simulink model "Class_task"  (R2020a)
settings: Solver=VariableStepAuto  StartTime=0.0  StopTime=10.0  RelTol=1e-3
settings Model: Creator=User  LastModifiedBy=User

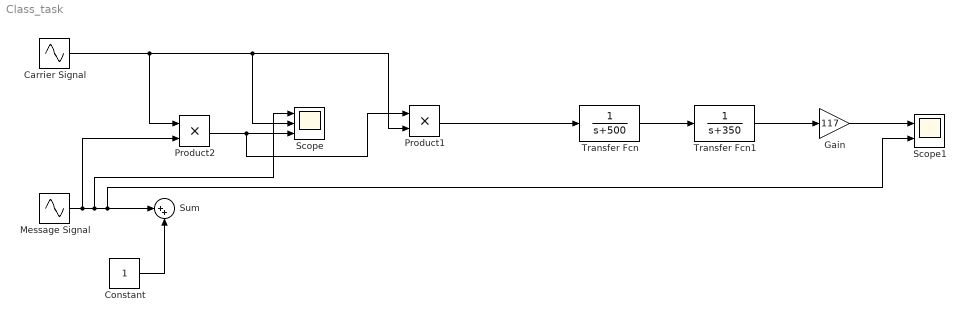
== system Class_task ==
  Carrier Signal : Sin  Amplitude=58  Frequency=2*pi*86  SampleTime=1/5000
  Constant : Constant
  Gain : Gain  Gain=117
  Message Signal : Sin  Amplitude=18  Frequency=2*pi*36  Phase=58  SampleTime=1/5000
  Product1 : Product
  Product2 : Product
  Scope : Scope  NumInputPorts=3
  Scope1 : Scope  NumInputPorts=2
  Sum : Sum  Inputs=|++
  Transfer Fcn : TransferFcn  Denominator=[1 500]
  Transfer Fcn1 : TransferFcn  Denominator=[1 350]
  wires:
  Constant/1 -> Sum/2
  Message Signal/1 -> Product2/2, Scope/1, Scope1/2, Sum/1
  Carrier Signal/1 -> Product1/2, Scope/2, Product2/1
  Product2/1 -> Product1/1, Scope/3
  Product1/1 -> Transfer Fcn/1
  Transfer Fcn/1 -> Transfer Fcn1/1
  Transfer Fcn1/1 -> Gain/1
  Gain/1 -> Scope1/1
